simulink model "F16_K_pqr2"  (R2023b)
settings: Solver=ode4  StartTime=0  StopTime=10  FixedStep=0.005  RelTol=1e-3  EnableMultiTasking=on
values from neighbouring files (symbols this model uses):
  C_rate = C([7:9 13],:)    [compare_lin_nonlin.m]    (also in plot_Kq_lin_nonlin.m; runsim_K_pqr.m)
  fc_rate = 1/2*ones(4,1)    [compare_lin_nonlin.m]    (also in plot_Kq_lin_nonlin.m; runsim_K_pqr.m)
  fi_rate = 1/4*ones(4,1)    [compare_lin_nonlin.m]    (also in plot_Kq_lin_nonlin.m; runsim_K_pqr.m)
  K_rate = 8*ones(4,1)    [compare_lin_nonlin.m]    (also in plot_Kq_lin_nonlin.m; runsim_K_pqr.m)
  X_trim = [501.999976668 0.0505473192089 -2.30406790676e-05 0.000102787556036 0.0505344970072 7.11881239542e-07 -0.000134428882921 -3.64533551716e-06 -1.91663482729e-05 0 0 0 ... (13 elements, 13x1)]    [trimcond.mat]
  xcg = 0.35    [trimcond.mat]
settings Model: PauseTimes=1.5  Creator=keviczky  LastModifiedBy=suvo
settings DataIOCC: Decimation=50  SaveFormat=Array  SignalLoggingSaveFormat=ModelDataLogs  ReturnWorkspaceOutputs=off  SignalLoggingName=sigsOut
settings OptimizationCC: BooleanDataType=off
settings DebuggingCC: SaveWithParameterizedLinksMsg=none  UnderspecifiedInitializationDetection=Classic  MergeDetectMultiDrivingBlocksExec=none  SignalResolutionControl=TryResolveAllWithWarning  MultiTaskDSMMsg=warning  MultiTaskCondExecSysMsg=none  UnconnectedInputMsg=warning  UnconnectedOutputMsg=warning  UnconnectedLineMsg=warning
settings HardwareCC: ProdBitPerPointer=32  ProdBitPerSizeT=32  ProdBitPerPtrDiffT=32  ProdLargestAtomicFloat=None  ProdIntDivRoundTo=Undefined  ProdEndianess=Unspecified  ProdWordSize=32  ProdHWDeviceType=32-bit Generic  TargetUnknown=on
settings ModelReferenceCC: PropagateSignalLabelsOutOfModel=off
settings GRTTargetCC: CombineOutputUpdateFcns=off  GRTInterface=on
settings ConfigComp: CovMetricSettings=dw  CovSaveCumulativeToWorkspaceVar=on  CovSaveSingleToWorkspaceVar=on

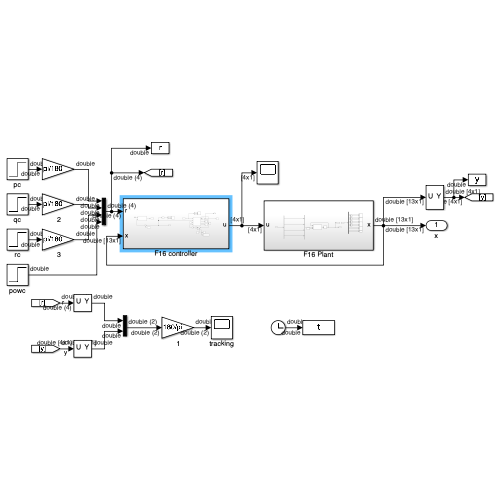
[thumbnail: Simulink's stored preview of the top-level diagram]
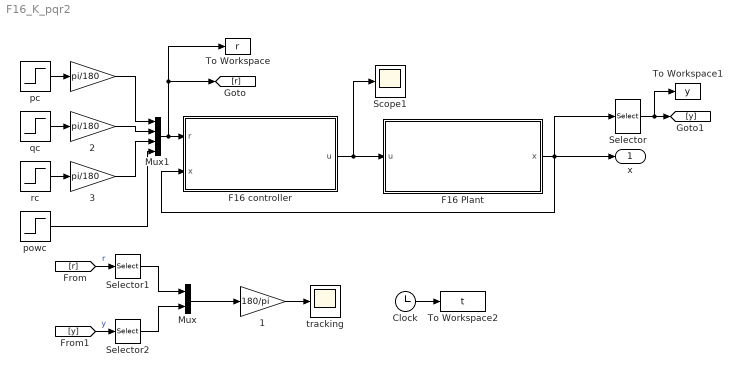
== system F16_K_pqr2 ==
  " " : Gain  Gain=pi/180
  " 1" : Gain  Gain=180/pi
  " 2" : Gain  Gain=pi/180
  " 3" : Gain  Gain=pi/180
  Clock : Clock
  F16 Plant : Subsystem
  F16 controller : Subsystem
  Mux : Mux  Inputs=2
  Mux1 : Mux
  Scope1 : Scope
  Selector : Selector  InputPortWidth=13  IndexOptions=Index vector (dialog)  Indices=[7:9 13]  OutputSizes=1
  Selector1 : Selector  InputPortWidth=4  IndexOptions=Index vector (dialog)  Indices=2  OutputSizes=1
  Selector2 : Selector  InputPortWidth=4  IndexOptions=Index vector (dialog)  Indices=2  OutputSizes=1
  To Workspace : ToWorkspace  VariableName=r  SampleTime=-1
  To Workspace1 : ToWorkspace  VariableName=y  SampleTime=-1
  To Workspace2 : ToWorkspace  VariableName=t  SampleTime=-1
  pc : Step  Time=0  After=0  SampleTime=0
  powc : Step  Time=0  After=0  SampleTime=0
  qc : Step  Time=0.1  SampleTime=0
  rc : Step  Time=0  After=0  SampleTime=0
  tracking : Scope
  x : Outport
  wires:
  pc/1 -> " "/1
  [r] -> Selector1/1  "r"
  [y] -> Selector2/1  "y"
  Mux/1 -> " 1"/1
  Selector/1 -> To Workspace1/1, [y]
  " 1"/1 -> tracking/1
  Clock/1 -> To Workspace2/1
  F16 Plant/1(x) -> F16 controller/2(x), Selector/1, x/1
  Mux1/1 -> [r], To Workspace/1, F16 controller/1(r)
  qc/1 -> " 2"/1
  rc/1 -> " 3"/1
  F16 controller/1(u) -> Scope1/1, F16 Plant/1(u)
  Selector1/1 -> Mux/1
  Selector2/1 -> Mux/2
  " "/1 -> Mux1/1
  " 2"/1 -> Mux1/2
  " 3"/1 -> Mux1/3
  powc/1 -> Mux1/4

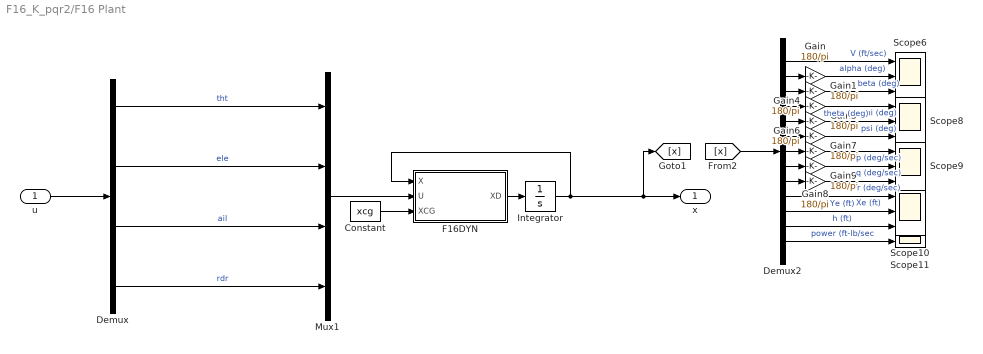
== system F16_K_pqr2/F16 Plant ==
  u : Inport
  Constant : Constant  Value=xcg
  Demux : Demux
  Demux2 : Demux  Outputs=13
  F16DYN : MATLAB Function  TreatAsAtomicUnit=on
  Gain{,1,4..9} (8 alike) : Gain  Gain=180/pi
  Integrator : Integrator  InitialCondition=X_trim
  Mux1 : Mux
  Scope{6,8..10} (4 alike) : Scope  NumInputPorts=3
  Scope11 : Scope
  x : Outport
  wires:
  Demux2/7 -> Gain7/1
  Demux2/11 -> Scope10/2  "Ye (ft)"
  Demux2/2 -> Gain/1
  Demux2/10 -> Scope10/1  "Xe (ft)"
  F16DYN/1(XD) -> Integrator/1
  Gain4/1 -> Scope8/1  "phi (deg)"
  Demux2/5 -> Gain5/1
  Gain6/1 -> Scope8/3  "psi (deg)"
  Gain/1 -> Scope6/2  "alpha (deg)"
  Demux2/8 -> Gain8/1
  Gain8/1 -> Scope9/2  "q (deg/sec)"
  Mux1/1 -> F16DYN/2(U)
  Gain9/1 -> Scope9/3  "r (deg/sec)"
  Demux2/6 -> Gain6/1
  Demux2/3 -> Gain1/1
  Demux2/12 -> Scope10/3  "h (ft)"
  Gain1/1 -> Scope6/3  "beta (deg)"
  Demux2/13 -> Scope11/1  "power (ft-lb/sec"
  Demux2/1 -> Scope6/1  "V (ft/sec)"
  Gain7/1 -> Scope9/1  "p (deg/sec)"
  Constant/1 -> F16DYN/3(XCG)
  [x] -> Demux2/1
  Demux2/9 -> Gain9/1
  Demux2/4 -> Gain4/1
  Gain5/1 -> Scope8/2  "theta (deg)"
  Demux/4 -> Mux1/4  "rdr"
  Demux/3 -> Mux1/3  "ail"
  Demux/2 -> Mux1/2  "ele"
  Demux/1 -> Mux1/1  "tht"
  Integrator/1 -> [x], x/1, F16DYN/1(X)
  u/1 -> Demux/1

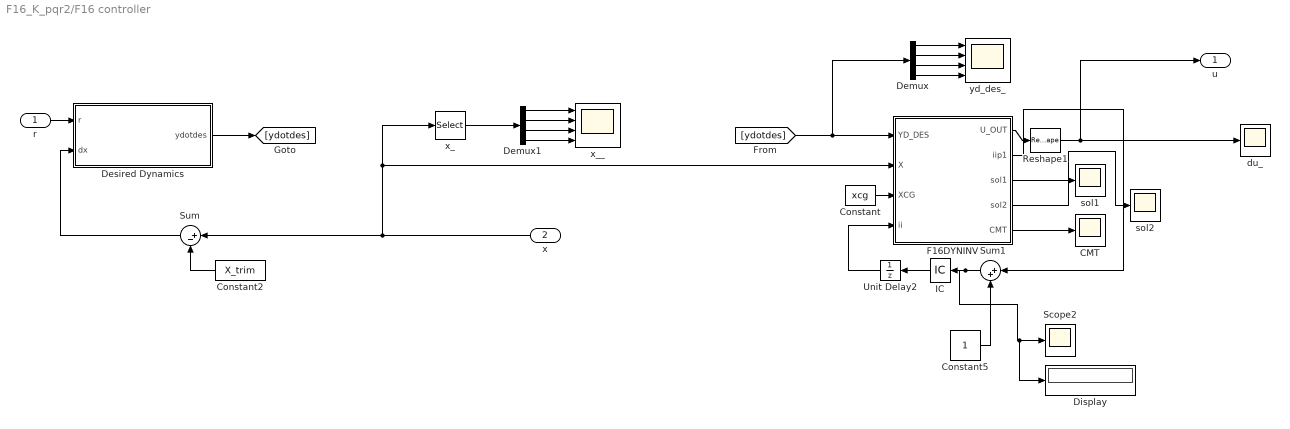
== system F16_K_pqr2/F16 controller ==
  r : Inport
  x : Inport  Port=2
  CMT : Scope
  Constant : Constant  Value=xcg
  Constant2 : Constant  Value=X_trim
  Constant5 : Constant
  Demux : Demux
  Demux1 : Demux
  Desired Dynamics : Subsystem
  Display : Display
  F16DYNINV : MATLAB Function  TreatAsAtomicUnit=on
  IC : InitialCondition
  Reshape1 : Reshape  OutputDimensionality=Column vector (2-D)
  Scope2 : Scope
  Sum : Sum  Inputs=|+-
  Sum1 : Sum  Inputs=|++
  Unit Delay2 : UnitDelay  SampleTime=-1  HasFrameUpgradeWarning=on
  du_ : Scope
  sol1 : Scope
  sol2 : Scope
  x_ : Selector  InputPortWidth=13  IndexOptions=Index vector (dialog)  Indices=[7 8 9 13]  OutputSizes=1
  x__ : Scope  NumInputPorts=4
  yd_des_ : Scope  NumInputPorts=4
  u : Outport
  wires:
  F16DYNINV/1(U_OUT) -> Reshape1/1
  Constant/1 -> F16DYNINV/3(XCG)
  r/1 -> Desired Dynamics/1(r)
  x/1 -> F16DYNINV/2(X), x_/1, Sum/1
  Reshape1/1 -> du_/1, u/1
  Desired Dynamics/1(ydotdes) -> [ydotdes]
  [ydotdes] -> Demux/1, F16DYNINV/1(YD_DES)
  Demux/1 -> yd_des_/1
  Demux/2 -> yd_des_/2
  Demux/3 -> yd_des_/3
  Demux/4 -> yd_des_/4
  F16DYNINV/2(iip1) -> Sum1/1
  Constant5/1 -> Sum1/2
  Sum1/1 -> Display/1, Scope2/1, IC/1
  IC/1 -> Unit Delay2/1
  Unit Delay2/1 -> F16DYNINV/4(ii)
  F16DYNINV/3(sol1) -> sol1/1
  F16DYNINV/5(CMT) -> CMT/1
  x_/1 -> Demux1/1
  Demux1/3 -> x__/3
  Demux1/4 -> x__/4
  Demux1/1 -> x__/1
  Demux1/2 -> x__/2
  F16DYNINV/4(sol2) -> sol2/1
  Sum/1 -> Desired Dynamics/2(dx)
  Constant2/1 -> Sum/2

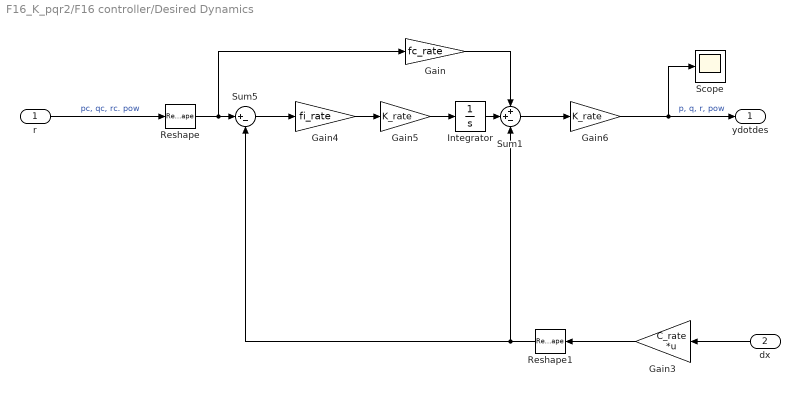
== system F16_K_pqr2/F16 controller/Desired Dynamics ==
  r : Inport
  dx : Inport  Port=2
  Gain : Gain  Gain=fc_rate
  Gain3 : Gain  Gain=C_rate  Multiplication=Matrix(K*u)
  Gain4 : Gain  Gain=fi_rate
  Gain5 : Gain  Gain=K_rate
  Gain6 : Gain  Gain=K_rate
  Integrator : Integrator  InitialCondition=[0; 0; 0; 0]
  Reshape : Reshape  OutputDimensionality=Column vector (2-D)
  Reshape1 : Reshape  OutputDimensionality=Column vector (2-D)
  Scope : Scope
  Sum1 : Sum  Inputs=++-
  Sum5 : Sum  Inputs=|+-
  ydotdes : Outport
  wires:
  Integrator/1 -> Sum1/2
  r/1 -> Reshape/1  "pc, qc, rc. pow"
  Sum1/1 -> Gain6/1
  Gain4/1 -> Gain5/1
  dx/1 -> Gain3/1
  Gain/1 -> Sum1/1
  Gain6/1 -> Scope/1, ydotdes/1  "p, q, r, pow"
  Gain5/1 -> Integrator/1
  Sum5/1 -> Gain4/1
  Gain3/1 -> Reshape1/1
  Reshape/1 -> Gain/1, Sum5/1
  Reshape1/1 -> Sum1/3, Sum5/2

== matlab function F16_K_pqr2/F16 controller/F16DYNINV ==
  data: YD_DES input; X input; XCG input; U_OUT output size=4; ii input; iip1 output; sol1 output; sol2 output; CMT output
function [U_OUT,iip1, sol1, sol2, CMT] = F16DYNINV(YD_DES,X,XCG,ii)
% f16 dynamics

% Author: Subhabrata Ganguli
%
% Ref: Stevens, Brian L.; Lewis, Frank L.; Johnson, Eric N.. 
% Aircraft Control and Simulation: Dynamics, 
% Controls Design, and Autonomous Systems. 
% Wiley.

U_OUT = zeros(4,1);

%% Parameters

IXX = 9496.0;
IYY = 55814.0;
IZZ = 63100.0;
IXZ =   982.0;

AXX = IXX;
AYY = IYY;
AZZ = IZZ;
AXZ = IXZ;

AXZS = AXZ^2;
XPQ  = AXZ * (AXX - AYY + AZZ);
GAM  = AXX * AZZ - AXZ^2;

XQR = AZZ * (AZZ - AYY) + AXZS;
ZPQ =(AXX-AYY) * AXX + AXZS;
YPR = AZZ - AXX;

WEIGHT = 25000.0;
GD = 32.174;
MASS = WEIGHT/GD;

S = 300;
B = 30;
CBAR = 11.32;
XCGR = 0.35;
HX = 160;
RTOD = 180/pi;

%% Assign State Variables

VT = X(1); 
ALPHA = X(2)*RTOD; 
BETA = X(3)*RTOD;
PHI = X(4); 
THETA = X(5); 
PSI = X(6);
P = X(7); 
Q = X(8); 
R = X(9); 
ALT = X(12); 
POW = X(13);

%% Air data computer and engine model

[TFAC, TEMP, RHO, AMACH, QBAR, PS ] = ADC(VT, ALT);

CPOW = PDOTINV(POW,YD_DES(4));
[THTL, sol1] = TGEARINV(CPOW);
T = THRUST(POW,ALT,AMACH);

QS    = QBAR * S; 
QSB   = QS * B; 
QHX   = Q*HX;

%% State varibles

CBTA  = cos(X(3)); 
U     = VT*cos(X(2))*CBTA;
V     = VT * sin(X(3)); 
W     = VT*sin(X(2))*CBTA;
STH   = sin(THETA); 
CTH   = cos(THETA);   
SPH   = sin(PHI);
CPH   = cos(PHI); 
SPSI  = sin(PSI);    
CPSI  = cos(PSI);
QS    = QBAR * S; 
QSB   = QS * B;        
RMQS  = QS/MASS;
GCTH  = GD * CTH; 
QSPH  = Q * SPH;

%% Forces

DUM   = (U*U + W*W);
AMAT = [ U  V  W;
        -W  0  U;
         0 VT  0];
BVEC = [VT*XD(1); DUM*XD(2); (DUM/CBTA)*XD(3) + V*XD(1)];

TMP = AMAT\BVEC;
UDOT = TMP(1);
VDOT = TMP(2);
WDOT = TMP(3);

CXT = ((UDOT - R*V + Q*W + GD*STH)*MASS - T)/QS;
AY = VDOT - P*W + R*U - GCTH * SPH;
AZ = WDOT - Q*U + P*V - GCTH * CPH;
CYT   = AY/RMQS; 
CZT   = AZ/RMQS;

%% Moments

PDOT_ = YD_DES(1);
QDOT_ = YD_DES(2);
RDOT_ = YD_DES(3);

ROLL = IXX*PDOT_ - IXZ*RDOT_ + (IZZ-IYY)*Q*R - IXZ*P*Q;
PITCH = IYY*QDOT_ - YPR*R*P + IXZ*(P^2-R^2) + R*HX;
YAW = -IXZ*PDOT_ + IZZ*RDOT_ + (IYY-IXX)*P*Q + IXZ*Q*R - QHX;

CLT = ROLL/QSB;
CMT = PITCH/(QS *CBAR);
CNT = YAW/QSB;

TVT = 0.5/VT; 
B2V = B*TVT; 
CQ = CBAR*Q*TVT;

D = DAMP(ALPHA);

CXT = CXT - (CQ * D(1));
CYT = CYT - (B2V * ( D(2)*R + D(3)*P ));
CZT = CZT - (CQ * D(4));
CLT = CLT - (B2V * ( D(5)*R + D(6)*P ));
CMT = CMT - (CQ * D(7) + CZT * (XCGR-XCG));
CNT = CNT - (B2V*(D(8)*R + D(9)*P) - CYT*(XCGR-XCG) * CBAR/B);

%% Look-up tables and component buildup
      
DLDA_OUT = DLDA(ALPHA,BETA);
DLDR_OUT = DLDR(ALPHA,BETA);
DNDA_OUT = DNDA(ALPHA,BETA);
DNDR_OUT = DNDR(ALPHA,BETA);

A1 = CL(ALPHA,BETA);
B1 = DLDA_OUT;
C1 = DLDR_OUT;
D1 = CLT;

A2 = CN(ALPHA,BETA);
B2 = DNDA_OUT;
C2 = DNDR_OUT;
D2 = CNT;

%DAIL1 = ((D1*B2-D2*B1) - (A1*B2-A2*B1))/(C1*B2-C2*B1)
%DRDR1 = ((D1*C2-D2*C1) - (A1*C2-A2*C1))/(B1*C2-B2*C1)

mat = [B1 C1;
        B2 C2];
vec = [(D1-A1); (D2-A2)];

inv = mat\vec;
DAIL = inv(1);
DRDR = inv(2);

[EL,sol2] = CMINV(CMT,ALPHA);
AIL = DAIL * 20.0; 
RDR = DRDR * 30.0;

U_OUT(1) = THTL;
U_OUT(2) = EL;
U_OUT(3) = AIL;
U_OUT(4) = RDR;

U_OUT = U_OUT(:);

% figure(1)
% plot(ii,CMT,'r*')
% hold on
% iip1 = ii;

end

== matlab function F16_K_pqr2/F16 Plant/F16DYN ==
  data: X input; U input; XD output; XCG input
function XD = F16DYN(X,U,XCG)
% f16 dynamics

% Author: Subhabrata Ganguli
%
% Ref: Stevens, Brian L.; Lewis, Frank L.; Johnson, Eric N.. 
% Aircraft Control and Simulation: Dynamics, 
% Controls Design, and Autonomous Systems. 
% Wiley.

%% Parameters

AXX = 9496.0;
AYY = 55814.0;
AZZ = 63100.0;
AXZ =   982.0;

AXZS = AXZ^2;
XPQ  = AXZ * (AXX - AYY + AZZ);
GAM  = AXX * AZZ - AXZ^2;

XQR = AZZ * (AZZ - AYY) + AXZS;
ZPQ =(AXX-AYY) * AXX + AXZS;
YPR = AZZ - AXX;

WEIGHT = 25000.0;
GD = 32.174;
MASS = WEIGHT/GD;

S = 300;
B = 30;
CBAR = 11.32;
XCGR = 0.35;
HX = 160;
RTOD = 180/pi;

%% Assign State and Control Variables

VT = X(1); 
ALPHA = X(2)*RTOD; 
BETA = X(3)*RTOD;
PHI = X(4); 
THETA = X(5); 
PSI = X(6);
P = X(7); 
Q = X(8); 
R = X(9); 
ALT = X(12); 
POW = X(13);

THTL = U(1);
EL = U(2);
AIL = U(3);
RDR = U(4);

XD = zeros(13,1);

%% Air data computer and engine model

[TFAC, TEMP, RHO, AMACH, QBAR, PS ] = ADC(VT, ALT);
CPOW = TGEAR(THTL);

XD(13) = PDOT(POW,CPOW);     
T = THRUST(POW,ALT,AMACH);

%% Look-up tables and component buildup

CXT = CX (ALPHA,EL);
CYT = CY (BETA,AIL,RDR);
CZT = CZ (ALPHA,BETA,EL);
      
DAIL= AIL/20.0; DRDR= RDR/30.0;

DLDA_OUT = DLDA(ALPHA,BETA);
DLDR_OUT = DLDR(ALPHA,BETA);
DNDA_OUT = DNDA(ALPHA,BETA);
DNDR_OUT = DNDR(ALPHA,BETA);

CLT = CL(ALPHA,BETA) + DLDA_OUT*DAIL + DLDR_OUT*DRDR;
CMT = CM(ALPHA,EL);
CNT = CN(ALPHA,BETA) + DNDA_OUT*DAIL ...
    + DNDR_OUT*DRDR;

%% Add damping derivatives

TVT = 0.5/VT; 
B2V = B*TVT; 
CQ = CBAR*Q*TVT;

D = DAMP(ALPHA);

CXT = CXT + CQ * D(1);
CYT = CYT + B2V * ( D(2)*R + D(3)*P );
CZT = CZT + CQ * D(4);
CLT = CLT + B2V * ( D(5)*R + D(6)*P );
CMT = CMT + CQ * D(7) + CZT * (XCGR-XCG);
CNT = CNT + B2V*(D(8)*R + D(9)*P) - CYT*(XCGR-XCG) * CBAR/B;

%% Get ready for state equations

CBTA  = cos(X(3)); 
U     = VT*cos(X(2))*CBTA;
V     = VT * sin(X(3)); 
W     = VT*sin(X(2))*CBTA;
STH   = sin(THETA); 
CTH   = cos(THETA);   
SPH   = sin(PHI);
CPH   = cos(PHI); 
SPSI  = sin(PSI);    
CPSI  = cos(PSI);
QS    = QBAR * S; 
QSB   = QS * B;        
RMQS  = QS/MASS;
GCTH  = GD * CTH; 
QSPH  = Q * SPH;
AY    = RMQS*CYT; 
AZ    = RMQS * CZT;

%% Force Equations

UDOT   = R*V - Q*W - GD*STH + (QS * CXT + T)/MASS;
VDOT   = P*W - R*U + GCTH * SPH + AY;
WDOT   = Q*U - P*V + GCTH * CPH + AZ;
    
DUM   = (U*U + W*W);
XD(1) = (U*UDOT + V*VDOT + W*WDOT)/VT;
XD(2) = (U*WDOT - W*UDOT) / DUM;
XD(3) = (VT*VDOT- V*XD(1)) * CBTA / DUM;

%% Kinematics

XD(4) = P + (STH/CTH)*(QSPH + R*CPH);
XD(5) = Q*CPH - R*SPH;
XD(6) = (QSPH + R*CPH)/CTH;

%% Moments

ROLL  = QSB*CLT;
PITCH = QS *CBAR*CMT;
YAW   = QSB*CNT;
PQ    = P*Q;
QR    = Q*R;
QHX   = Q*HX;
XD(7) = ( XPQ*PQ - XQR*QR + AZZ*ROLL + AXZ*(YAW + QHX) )/GAM;
XD(8) = ( YPR*P*R - AXZ*(P^2 - R^2) + PITCH - R*HX )/AYY;
XD(9) = ( ZPQ*PQ - XPQ*QR + AXZ*ROLL + AXX*(YAW + QHX) )/GAM;

end
